simulink model "sist_cont_dt_smith_diff"  (Simulink 7.2)
settings: Solver=ode45  StartTime=0.0  StopTime=10.0  RelTol=1e-3
libraries: simulink_extras x1
settings Model: Creator=CrisGC  LastModifiedBy=CrisGC

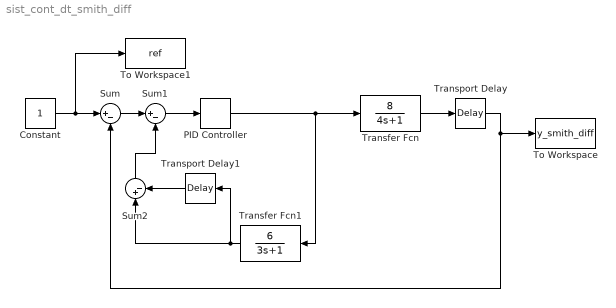
== system sist_cont_dt_smith_diff ==
  Constant : Constant  OutDataType=sfix(16)  OutScaling=2^0
  PID Controller : simulink_extras/Additional Linear/PID Controller  SystemSampleTime=-1  P=1  I=0.2  D=0
  Sum : Sum  Inputs=|+-  OutDataType=sfix(16)  OutScaling=2^0
  Sum1 : Sum  Inputs=|+-  OutDataType=sfix(16)  OutScaling=2^0
  Sum2 : Sum  Orientation=up  Inputs=|+-  OutDataType=sfix(16)  OutScaling=2^0
  To Workspace : ToWorkspace  VariableName=y_smith_diff  SampleTime=-1  SaveFormat=Array
  To Workspace1 : ToWorkspace  VariableName=ref  SampleTime=-1  SaveFormat=Array
  Transfer Fcn : TransferFcn  Numerator=[8]  Denominator=[4 1]
  Transfer Fcn1 : TransferFcn  Orientation=left  Numerator=[6]  Denominator=[3 1]
  Transport Delay : TransportDelay
  Transport Delay1 : TransportDelay  Orientation=left
  wires:
  Constant/1 -> Sum/1, To Workspace1/1
  PID Controller/1 -> Transfer Fcn/1, Transfer Fcn1/1
  Transfer Fcn/1 -> Transport Delay/1
  Transport Delay/1 -> Sum/2, To Workspace/1
  Sum/1 -> Sum1/1
  Sum1/1 -> PID Controller/1
  Transfer Fcn1/1 -> Sum2/1, Transport Delay1/1
  Transport Delay1/1 -> Sum2/2
  Sum2/1 -> Sum1/2
